simulink model "modelnew"  (R2015a)
settings: Solver=ode15s  SolverMode=SingleTasking  StartTime=0.0  StopTime=8  RelTol=1e-3
undefined symbols (not defined in the file): a, b, k1z, k2z, L1, L2, M1, M2, q1f, qf2, R1, r1z, R2, r2z
libraries: aerolibutil x2
settings Model: Creator=User  LastModifiedBy=User
settings DataIOCC: SignalLoggingSaveFormat=ModelDataLogs
settings OptimizationCC: BlockReduction=off  BooleanDataType=off
settings DebuggingCC: SaveWithParameterizedLinksMsg=none  UnderspecifiedInitializationDetection=Classic  MergeDetectMultiDrivingBlocksExec=none  SignalResolutionControl=TryResolveAllWithWarning  MultiTaskDSMMsg=warning  MultiTaskCondExecSysMsg=none  StateNameClashWarn=warning
settings HardwareCC: TargetUnknown=on

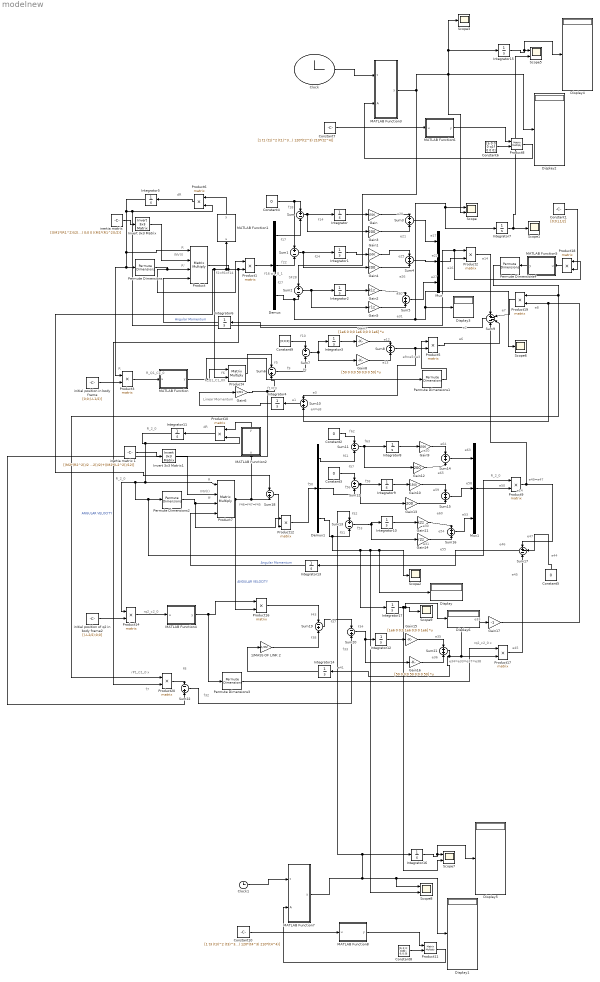
== system modelnew ==
  note: e33
  note: e41
  note: e8
  note: e36
  note: e35
  note: rq2_c2_0 x
  note: f34
  note: f33
  note: f32
  note: f8
  note: f7
  note: rP1_C1_0 x
  note: f38
  note: e1
  note: e3
  note: e4=e8
  note: e7
  note: e44
  note: e45
  note: e45
  note: e34=e33=e37=e38
  note: f37
  note: f43
  note: rq2_c2_0
  note: e47
  note: R_2_0
  note: R_2_0
  note: e49=e47
  note: R_2_0
  note: e50
  note: e53
  note: e58
  note: e63
  note: e55
  note: e54
  note: e60
  note: e59
  note: e65
  note: e64
  note: f63
  note: f58
  note: f57
  note: f53
  note: f51
  note: f56
  note: f62
  note: f52
  note: f61
  note: f50
  note: f9
  note: f6
  note: f2=f6=f14
  note: Linear Momentum
  note: e2
  note: dR
  note: f16
      | w1_0_1
  note: R
  note: R'
  note: R
  note: e6
  note: f5
  note: R_Q1_C1_0X
  note: e9=e5=e3
  note: e13
  note: e12
  note: f10
  note: f9
  note: f1=f3
  note: R_Q1_C1_0
  note: e16
  note: e27
  note: e22
  note: e17
  note: SF28
  note: f18
  note: e14
  note: e31
  note: e30
  note: e26
  note: e25
  note: e21
  note: e20
  note: f27
  note: f22
  note: f17
  note: f24
  note: f14
  note: INV(I)
  note: f46=f47=f45
  note: e46
  note: dR
  note: R'
  note: R
  note: e14
  note: e31
  note: e30
  note: e20
  note: INV(I)
  1/MASS OF LINK 2 : Gain  Gain=1/M2
  Clock : Clock
      settings: Decimation=2
  Clock1 : Clock
  Constant1 : Constant  Value=[0;0;L1/2]
  Constant10 : Constant  Value=[1 t3 (t3)^2 (t3)^3 (t3)^4 (t3)^5 (t3)^6 (t3)^7; 0 1 2*(t3) 3*((t3)^2) 4*((t3)^3) 5*((t3)^4) 6*((t3)^5) 7*((t3)^6); 0 0 2 6*(t3) 12*((t3)^2) 20*((t3)^3) 30*((t3)^4) 42*((t3)^5); 0 0 0 6 24*(t3) 60*((t3)^2) 120*((t3)^3) 210*((t3)^4); 1 t4 t4^2 t4^3 t4^4 t4^5 t4^6 t4^7; 0 1 2*t4 3*(t4^2) 4*(t4^3) 5*(t4^4) 6*(t4^5) 7*(t4^6);0 0 2 6*t4 12*(t4^2) 20*(t4^3) 30*(t4^4) 42*(t4^5);0 0 0 6 24*t4 60*(t4^2) 120*(t4^3) 210*(t4^4)]
  Constant{2..5} (4 alike) : Constant  Value=0
  Constant6 : Constant  Value=[a 0 0 0 q1f 0 0 0]
  Constant7 : Constant  Value=[1 t1 (t1)^2 (t1)^3 (t1)^4 (t1)^5 (t1)^6 (t1)^7; 0 1 2*(t1) 3*((t1)^2) 4*((t1)^3) 5*((t1)^4) 6*((t1)^5) 7*((t1)^6); 0 0 2 6*(t1) 12*((t1)^2) 20*((t1)^3) 30*((t1)^4) 42*((t1)^5); 0 0 0 6 24*(t1) 60*((t1)^2) 120*((t1)^3) 210*((t1)^4); 1 t2 t2^2 t2^3 t2^4 t2^5 t2^6 t2^7; 0 1 2*t2 3*(t2^2) 4*(t2^3) 5*(t2^4) 6*(t2^5) 7*(t2^6);0 0 2 6*t2 12*(t2^2) 20*(t2^3) 30*(t2^4) 42*(t2^5);0 0 0 6 24*t2 60*(t2^2) 120*(t2^3) 210*(t2^4)]
  Constant8 : Constant  Value=[b; 0; 0; 0;qf2 ; 0; 0; 0]
  Constant9 : Constant  Value=[0;0;0]  VectorParams1D=off
  Demux : Demux  Outputs=3
  Demux1 : Demux  Outputs=3
  Display{,1..6} (7 alike) : Display
      Display1 settings: Decimation=2
  Gain{,1,9..10} (4 alike) : Gain  Gain=1500
  Gain11 : Gain  Gain=k2z
  Gain{3..4,12..13} (4 alike) : Gain  Gain=200
  Gain14 : Gain  Gain=r2z
  Gain15 : Gain  Gain=[1e6 0 0;0 1e6 0;0 0 1e6]  Multiplication=Matrix(K*u)
  Gain16 : Gain  Gain=[50 0 0;0 50 0;0 0 50]  Multiplication=Matrix(K*u)
  Gain17 : Gain  Gain=-1
  Gain2 : Gain  Gain=k1z
  Gain5 : Gain  Gain=r1z
  Gain6 : Gain  Gain=1/M1
  Gain7 : Gain  Gain=[1e6 0 0;0 1e6 0;0 0 1e6]  Multiplication=Matrix(K*u)
  Gain8 : Gain  Gain=[50 0 0;0 50 0;0 0 50]  Multiplication=Matrix(K*u)
  Integrator{,1..3,7..10,12,15} (10 alike) : Integrator
  Integrator11 : Integrator  InitialCondition=[cos(a) -sin(a) 0;sin(a) cos(a) 0;0 0 1]*[cos(b) -sin(b) 0;0 0 -1;sin(b) cos(b) 0]
  Integrator{4,6,13..14} (4 alike) : Integrator  InitialCondition=[0;0;0]
  Integrator16 : Integrator  InitialCondition=-0.3490
  Integrator17 : Integrator  InitialCondition=-0.3490
  Integrator5 : Integrator  InitialCondition=[cos(a) -sin(a) 0;sin(a) cos(a) 0;0 0 1]
  Invert 3x3 Matrix : aerolibutil/Invert  3x3 Matrix
  Invert 3x3 Matrix1 : aerolibutil/Invert  3x3 Matrix
  MATLAB Function : MATLAB Function  TreatAsAtomicUnit=on
  MATLAB Function1 : MATLAB Function  TreatAsAtomicUnit=on
  MATLAB Function2 : MATLAB Function  TreatAsAtomicUnit=on
  MATLAB Function3 : MATLAB Function  TreatAsAtomicUnit=on
  MATLAB Function4 : MATLAB Function  TreatAsAtomicUnit=on
  MATLAB Function5 : MATLAB Function  TreatAsAtomicUnit=on
  MATLAB Function6 : MATLAB Function  TreatAsAtomicUnit=on
  MATLAB Function7 : MATLAB Function  TreatAsAtomicUnit=on
  MATLAB Function8 : MATLAB Function  TreatAsAtomicUnit=on
  Mux : Mux  Inputs=3
  Mux1 : Mux  Inputs=3
  Permute Dimensions{,1..4} (5 alike) : PermuteDimensions
  Product : Product  Inputs=4  Multiplication=Matrix(*)
  Product{1..6,8..12,14,16..20} (17 alike) : Product  Multiplication=Matrix(*)
  Product7 : Product  Inputs=4  Multiplication=Matrix(*)
  Scope{,5,7..8} (4 alike) : Scope  NumInputPorts=2
      Scope settings: YMin=-125~-5  YMax=225~5  SaveName=ScopeData2
      Scope5 settings: TimeRange=5  YMin=-5~-5  YMax=5~5  SaveName=ScopeData5
      Scope7 settings: YMin=-5~-5  YMax=5~5  SaveName=ScopeData7
      Scope8 settings: YMin=-5~-5  YMax=5~5  SaveName=ScopeData8
  Scope{1..3,6,9} (5 alike) : Scope
      Scope1 settings: YMin=0.205  YMax=0.226
      Scope2 settings: YMin=-90  YMax=80  SaveName=ScopeData3
      Scope3 settings: YMin=0.162  YMax=0.1675
      Scope6 settings: TimeRange=0.3076710970924061  YMin=-950  YMax=-700  SaveName=ScopeData6
      Scope9 settings: YMin=-90  YMax=80  SaveName=ScopeData9
  Sum{,1..2,7,11..13} (7 alike) : Sum  Inputs=+-
  Sum{3..5,8,10,14..16,21} (9 alike) : Sum
  Sum17 : Sum  Inputs=+--
  Sum{6,18..20,22} (5 alike) : Sum  Inputs=-+
  Sum9 : Sum  Inputs=+---
  "inertia matrix " : Constant  Value=[((M1*(R1^2))/2)+((M1*(L1^2))/12) 0 0;0 ((M1*(R1^2))/2)+((M1*(L1^2))/12) 0;0 0 ((M1*(R1^2))/2)]  VectorParams1D=off
  inertia matrix 1 : Constant  Value=[(M2*(R2^2))/2 0 0;0 ((M2*(R2^2))/2)+((M2*(L2^2))/12) 0;0 0 ((M2*(R2^2))/2)+((M2*(L2^2))/12)]  VectorParams1D=off
  initial position in body frame : Constant  Value=[0;0;(-L1/2)]
  initial position of q2 in body frame2 : Constant  Value=[(-L2/2);0;0]
  wires:
  Permute Dimensions/1 -> Product1/1, Product/3
  Product/1 -> Sum18/1, Product4/2, MATLAB Function1/1(u), Product20/2, Product1/2  "ANGULAR VELOCITY"
  "inertia matrix "/1 -> Invert 3x3 Matrix/1
  Invert 3x3 Matrix/1 -> Product/2
  Product1/1 -> Demux/1
  Demux/1 -> Sum/2
  Constant4/1 -> Sum1/1, Sum/1
  Demux/2 -> Sum1/2
  Sum1/1 -> Gain4/1, Integrator1/1
  Sum/1 -> Gain3/1, Integrator/1
  Demux/3 -> Display3/1, Scope6/1, Integrator7/1, Scope/1, Sum2/2
  Sum2/1 -> Gain5/1, Integrator2/1
  Integrator/1 -> Gain/1
  Integrator2/1 -> Gain2/1
  Integrator1/1 -> Gain1/1
  Gain/1 -> Sum3/1
  Gain3/1 -> Sum3/2
  Gain1/1 -> Sum4/1
  Gain4/1 -> Sum4/2
  Gain2/1 -> Sum5/1
  Gain5/1 -> Sum5/2
  Sum3/1 -> Mux/1
  Sum4/1 -> Mux/2
  Sum5/1 -> Mux/3
  Mux/1 -> Product2/2
  Product2/1 -> Sum9/1
  initial position in body frame/1 -> Product3/2
  Product3/1 -> MATLAB Function/1(u)
  MATLAB Function/1(y) -> Permute Dimensions1/1, Product4/1
  Product4/1 -> Sum6/1
  Gain6/1 -> Sum22/2, Sum6/2
  Sum6/1 -> Sum7/2
  Constant9/1 -> Sum7/1
  Sum7/1 -> Integrator3/1, Gain8/1
  Gain7/1 -> Sum8/1
  Gain8/1 -> Sum8/2
  Integrator3/1 -> Gain7/1
  Sum8/1 -> Sum10/1, Product5/2
  Permute Dimensions1/1 -> Product5/1
  Product5/1 -> Sum9/3
  MATLAB Function1/1(y) -> Product6/1
  Product6/1 -> Integrator5/1
  Integrator5/1 -> Product18/1, Product2/1, Product6/2, Product3/1, Permute Dimensions/1, Product/1
  Integrator4/1 -> Gain6/1
  Sum9/1 -> Integrator6/1
  Integrator6/1 -> Product/4  "Angular Momentum"
  Integrator7/1 -> Scope5/2, Scope1/1
  Sum10/1 -> Integrator4/1
  Product7/1 -> Product16/2, MATLAB Function2/1(u), Sum18/2  "ANGULAR VELOCITY"
  inertia matrix 1/1 -> Invert 3x3 Matrix1/1
  Invert 3x3 Matrix1/1 -> Product7/2
  Demux1/1 -> Sum11/2
  Demux1/2 -> Sum12/2
  Sum12/1 -> Gain13/1, Integrator9/1
  Demux1/3 -> Scope8/2, Display/1, Scope2/1, Integrator17/1, Sum13/2
  Sum13/1 -> Gain14/1, Integrator10/1
  Integrator8/1 -> Gain9/1
  Integrator10/1 -> Gain11/1
  Integrator9/1 -> Gain10/1
  Gain9/1 -> Sum14/1
  Gain12/1 -> Sum14/2
  Gain10/1 -> Sum15/1
  Gain11/1 -> Sum16/1
  Gain14/1 -> Sum16/2
  Sum14/1 -> Mux1/1
  Sum15/1 -> Mux1/2
  Sum16/1 -> Mux1/3
  MATLAB Function2/1(y) -> Product10/1
  Product10/1 -> Integrator11/1
  Sum17/1 -> Integrator13/1
  Integrator13/1 -> Product7/4  "Angular Momentum"
  Constant2/1 -> Sum11/1
  Sum11/1 -> Gain12/1, Integrator8/1
  Sum18/1 -> Product12/2
  Gain13/1 -> Sum15/2
  Constant3/1 -> Sum12/1
  Mux1/1 -> Product9/2
  Integrator11/1 -> Product9/1, Permute Dimensions2/1, Product14/1, Product7/1, Product10/2
  Permute Dimensions2/1 -> Product12/1, Product7/3
  Product12/1 -> Demux1/1
  initial position of q2 in body frame2/1 -> Product14/2
  Product14/1 -> MATLAB Function4/1(u)
  MATLAB Function4/1(y) -> Permute Dimensions3/1, Product16/1
  Product16/1 -> Sum19/1
  1/MASS OF LINK 2/1 -> Sum19/2
  Sum19/1 -> Sum20/1
  Sum22/1 -> Sum20/2
  Sum20/1 -> Integrator12/1, Gain16/1
  Integrator12/1 -> Gain15/1
  Gain15/1 -> Sum21/1
  Gain16/1 -> Sum21/2
  Permute Dimensions3/1 -> Product17/1
  Product17/1 -> Sum17/3
  Constant5/1 -> Sum17/2
  Product18/1 -> MATLAB Function5/1(u)
  MATLAB Function5/1(y) -> Permute Dimensions4/1
  Permute Dimensions4/1 -> Product20/1, Product19/1
  Product19/1 -> Sum9/2
  Sum21/1 -> Gain17/1, Product17/2, Integrator14/1
  Integrator14/1 -> 1/MASS OF LINK 2/1
  Product20/1 -> Sum22/1
  Product9/1 -> Sum17/1, Sum9/4
  Gain17/1 -> Sum10/2, Product19/2
  Constant1/1 -> Product18/2
  Clock/1 -> MATLAB Function3/1(t)
  Constant6/1 -> Product8/2
  Constant7/1 -> MATLAB Function6/1(u)
  MATLAB Function6/1(y) -> Product8/1
  Product8/1 -> MATLAB Function3/2(A)
  Integrator15/1 -> Display4/1, Scope5/1
  Clock1/1 -> MATLAB Function7/1(t)
  MATLAB Function7/1(y) -> Scope8/1, Display1/1, Integrator16/1, Sum13/1
  Constant8/1 -> Product11/2
  Constant10/1 -> MATLAB Function8/1(u)
  MATLAB Function8/1(y) -> Product11/1
  Product11/1 -> MATLAB Function7/2(A)
  Integrator16/1 -> Display5/1, Scope7/1
  Integrator17/1 -> Scope7/2, Display6/1, Scope9/1
  MATLAB Function3/1(y) -> Sum2/1, Scope/2, Integrator15/1, Scope3/1, Display2/1

== matlab function modelnew/MATLAB Function1 ==
  data: u input; y output
function y = fcn(u)
%#codegen

y = [0 -u(3) u(2);u(3) 0 -u(1); -u(2) u(1) 0];

== matlab function modelnew/MATLAB Function ==
  data: u input; y output
function y = fcn(u)
%#codegen

y = [0 -u(3) u(2);u(3) 0 -u(1); -u(2) u(1) 0];

== matlab function modelnew/MATLAB Function2 ==
  data: u input; y output
function y = fcn(u)
%#codegen

y = [0 -u(3) u(2);u(3) 0 -u(1); -u(2) u(1) 0];

== matlab function modelnew/MATLAB Function3 ==
  data: t input; y output; A input
function y = fcn(t,A)
%#codegen

y=A(2,1)+ 2*A(3,1)*t+ 3*A(4,1)*t^2 + 4*A(5,1)*t^3 + 5*A(6,1)*t^4 + 6*A(7,1)*t^5 + 7*A(8,1)*t^6;

== matlab function modelnew/MATLAB Function4 ==
  data: u input; y output
function y = fcn(u)
%#codegen

y = [0 -u(3) u(2);u(3) 0 -u(1); -u(2) u(1) 0];

== matlab function modelnew/MATLAB Function5 ==
  data: u input; y output
function y = fcn(u)
%#codegen

y = [0 -u(3) u(2);u(3) 0 -u(1); -u(2) u(1) 0];

== matlab function modelnew/MATLAB Function6 ==
  data: u input; y output
function y = fcn(u)
%#codegen

y = inv(u);

== matlab function modelnew/MATLAB Function7 ==
  data: t input; y output; A input
function y = fcn(t,A)
%#codegen

y=A(2,1)+ 2*A(3,1)*t+ 3*A(4,1)*t^2 + 4*A(5,1)*t^3 + 5*A(6,1)*t^4 + 6*A(7,1)*t^5 + 7*A(8,1)*t^6;

== matlab function modelnew/MATLAB Function8 ==
  data: u input; y output
function y = fcn(u)
%#codegen

y = inv(u);
